simulink model "teste"  (R2012b)
settings: Solver=ode3  StartTime=0.0  StopTime=0.2  FixedStep=1e-6  RelTol=1e-6
undefined symbols (not defined in the file): J, Kd, Ke, Kt, L, P, R
libraries: simulink x40
settings Model: BufferReuse=off  Creator=Juliano  LastModifiedBy=Juliano
settings OptimizationCC: OptimizeBlockIOStorage=off  BufferReuse=off  ExpressionFolding=off  LocalBlockOutputs=off
settings DebuggingCC: SignalInfNanChecking=error  IntegerOverflowMsg=error  ParameterPrecisionLossMsg=none

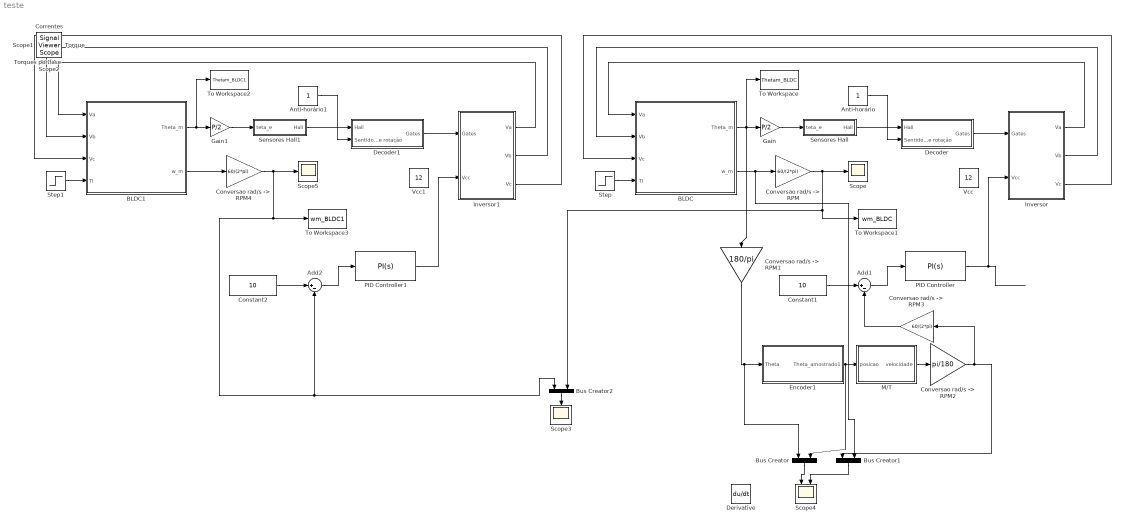
== system teste ==
  Add1 : Sum  Inputs=|+-
  Add2 : Sum  Inputs=|+-
  Anti-horário : Constant
  Anti-horário1 : Constant
  BLDC : Subsystem
  BLDC1 : Subsystem
  Bus Creator : BusCreator  Inputs=2
  Bus Creator1 : BusCreator  Inputs=2
  Bus Creator2 : BusCreator  Inputs=2
  Constant1 : Constant  Value=10
  Constant2 : Constant  Value=10
  "Conversao rad/s -> RPM" : Gain  Gain=60/(2*pi)
  "Conversao rad/s -> RPM1" : Gain  Gain=180/pi
  "Conversao rad/s -> RPM2" : Gain  Gain=pi/180
  "Conversao rad/s -> RPM3" : Gain  Gain=60/(2*pi)
  "Conversao rad/s -> RPM4" : Gain  Gain=60/(2*pi)
  Decoder : Subsystem
  Decoder1 : Subsystem
  Derivative : Derivative
  Encoder1 : Subsystem  mask{Nr=180}
      mask prompts: Nr "Número de pulsos por revolução"
  Gain : Gain  Gain=P/2
  Gain1 : Gain  Gain=P/2
  Inversor : Subsystem
  Inversor1 : Subsystem
  M/T : Subsystem  mask{Ts=0.01/4}
      mask prompts: Ts "Sampling time"
  PID Controller : simulink/Continuous/PID Controller  Controller=PI  TimeDomain=Continuous-time  SampleTime=1  IntegratorMethod=Forward Euler  FilterMethod=Forward Euler  Form=Parallel  P=0.0147690941731554  I=1.64756402232112  D=0  N=100  InitialConditionSource=internal  InitialConditionForIntegrator=8.9768  InitialConditionForFilter=0  ExternalReset=none  ZeroCross=off  LimitOutput=on  UpperSaturationLimit=12  LowerSaturationLimit=-12  LinearizeAsGain=off  AntiWindupMode=none  Kb=1  TrackingMode=off  Kt=1  PParamMin=[ ]  PParamMax=[ ]  IParamMin=[ ]  IParamMax=[ ]  DParamMin=[ ]  DParamMax=[ ]  NParamMin=[ ]  NParamMax=[ ]  KbParamMin=[ ]  KbParamMax=[ ]  KtParamMin=[ ]  KtParamMax=[ ]  POutMin=[ ]  POutMax=[ ]  IOutMin=[ ]  IOutMax=[ ]  DOutMin=[ ]  DOutMax=[ ]  NOutMin=[ ]  NOutMax=[ ]  KbOutMin=[ ]  KbOutMax=[ ]  KtOutMin=[ ]  KtOutMax=[ ]  IntegratorOutMin=[ ]  IntegratorOutMax=[ ]  FilterOutMin=[ ]  FilterOutMax=[ ]  SumOutMin=[ ]  SumOutMax=[ ]  SumI1OutMin=[ ]  SumI1OutMax=[ ]  SumI2OutMin=[ ]  SumI2OutMax=[ ]  SumI3OutMin=[ ]  SumI3OutMax=[ ]  SumDOutMin=[ ]  SumDOutMax=[ ]  SaturationOutMin=[ ]  SaturationOutMax=[ ]  IntegratorContinuousStateAttributes=''  IntegratorStateMustResolveToSignalObject=off  IntegratorRTWStateStorageClass=Auto  FilterContinuousStateAttributes=''  FilterStateMustResolveToSignalObject=off  FilterRTWStateStorageClass=Auto
  PID Controller1 : simulink/Continuous/PID Controller  Controller=PI  TimeDomain=Continuous-time  SampleTime=1  IntegratorMethod=Forward Euler  FilterMethod=Forward Euler  Form=Parallel  P=0.0147690941731554  I=1.64756402232112  D=0  N=100  InitialConditionSource=internal  InitialConditionForIntegrator=8.9768  InitialConditionForFilter=0  ExternalReset=none  ZeroCross=off  LimitOutput=on  UpperSaturationLimit=12  LowerSaturationLimit=-12  LinearizeAsGain=off  AntiWindupMode=none  Kb=1  TrackingMode=off  Kt=1  PParamMin=[ ]  PParamMax=[ ]  IParamMin=[ ]  IParamMax=[ ]  DParamMin=[ ]  DParamMax=[ ]  NParamMin=[ ]  NParamMax=[ ]  KbParamMin=[ ]  KbParamMax=[ ]  KtParamMin=[ ]  KtParamMax=[ ]  POutMin=[ ]  POutMax=[ ]  IOutMin=[ ]  IOutMax=[ ]  DOutMin=[ ]  DOutMax=[ ]  NOutMin=[ ]  NOutMax=[ ]  KbOutMin=[ ]  KbOutMax=[ ]  KtOutMin=[ ]  KtOutMax=[ ]  IntegratorOutMin=[ ]  IntegratorOutMax=[ ]  FilterOutMin=[ ]  FilterOutMax=[ ]  SumOutMin=[ ]  SumOutMax=[ ]  SumI1OutMin=[ ]  SumI1OutMax=[ ]  SumI2OutMin=[ ]  SumI2OutMax=[ ]  SumI3OutMin=[ ]  SumI3OutMax=[ ]  SumDOutMin=[ ]  SumDOutMax=[ ]  SaturationOutMin=[ ]  SaturationOutMax=[ ]  IntegratorContinuousStateAttributes=''  IntegratorStateMustResolveToSignalObject=off  IntegratorRTWStateStorageClass=Auto  FilterContinuousStateAttributes=''  FilterStateMustResolveToSignalObject=off  FilterRTWStateStorageClass=Auto
  Scope : Scope
      settings: TimeRange=0.5  YMin=1100  YMax=3400
  Scope3 : Scope
      settings: TickLabels=on  ShowLegends=on  TimeRange=0.25  YMin=-750  YMax=4250
  Scope4 : Scope  NumInputPorts=2
      settings: TickLabels=on  YMin=900~-75  YMax=2800~425  SaveName=ScopeData7
  Scope5 : Scope
      settings: TimeRange=0.5  YMin=1100  YMax=3400  SaveName=ScopeData9
  Sensores Hall : Subsystem  AncestorBlock=spsPMSynchronousMachineModel/Discrete Trapezoidal/Hall effect sensor
  Sensores Hall1 : Subsystem  AncestorBlock=spsPMSynchronousMachineModel/Discrete Trapezoidal/Hall effect sensor
  Step : Step  Time=0.2  After=0*2e-3  SampleTime=0
  Step1 : Step  Time=0.2  After=0*2e-3  SampleTime=0
  To Workspace : ToWorkspace  VariableName=Thetam_BLDC  SampleTime=-1  SaveFormat=Timeseries
  To Workspace1 : ToWorkspace  VariableName=wm_BLDC  SampleTime=-1  SaveFormat=Timeseries
  To Workspace2 : ToWorkspace  VariableName=Thetam_BLDC1  SampleTime=-1  SaveFormat=Timeseries
  To Workspace3 : ToWorkspace  VariableName=wm_BLDC1  SampleTime=-1  SaveFormat=Timeseries
  Vcc : Constant  Value=12
  Vcc1 : Constant  Value=12
  Correntes : SignalViewerScope  IOType=viewer  NumInputPorts=3  ZoomMode=yonly  RefreshTime=0.035000
      settings: YMin=-5~-5~-5  YMax=5~5~5
  FCEMs : SignalViewerScope  IOType=viewer  NumInputPorts=3  ZoomMode=xonly  RefreshTime=0.035000
      settings: YMin=-5~-5~-5  YMax=5~5~5  SaveName=ScopeData2
  Scope1 : SignalViewerScope  IOType=viewer  RefreshTime=0.035000
      settings: SaveName=ScopeData3
  Scope2 : SignalViewerScope  IOType=viewer  RefreshTime=0.035000
      settings: SaveName=ScopeData4
  Torque : SignalViewerScope  IOType=viewer  ZoomMode=xonly  RefreshTime=0.035000
      settings: SaveToWorkspace=on  SaveName=Torque
  Torques por fase : SignalViewerScope  IOType=viewer  NumInputPorts=3  ZoomMode=xonly  RefreshTime=0.035000
      settings: YMin=-5~-5~-5  YMax=5~5~5
  wires:
  Gain/1 -> Sensores Hall/1(teta_e)
  Sensores Hall/1(Hall) -> Decoder/1("Hall ")
  Decoder/1(Gates) -> Inversor/1(Gates)
  Anti-horário/1 -> Decoder/2(Sentido de rotação)
  Step/1 -> BLDC/4(Tl)
  Inversor/1(Va) -> BLDC/1(Va)
  Inversor/2(Vb) -> BLDC/2(Vb)
  Inversor/3(Vc) -> BLDC/3(Vc)
  BLDC/2(w_m) -> Bus Creator1/2, "Conversao rad/s -> RPM"/1
  "Conversao rad/s -> RPM"/1 -> Bus Creator2/2, To Workspace1/1, Scope/1
  Constant1/1 -> Add1/1
  Add1/1 -> PID Controller/1
  Bus Creator/1 -> Scope4/1
  Bus Creator1/1 -> Scope4/2
  Encoder1/1(Theta_amostrado1) -> M/T/1(posicao), Bus Creator/2
  PID Controller/1 -> Inversor/2(Vcc)
  BLDC/1(Theta_m) -> "Conversao rad/s -> RPM1"/1, Gain/1, To Workspace/1
  M/T/1(velocidade) -> "Conversao rad/s -> RPM2"/1
  "Conversao rad/s -> RPM1"/1 -> Bus Creator/1, Encoder1/1(Theta)
  "Conversao rad/s -> RPM2"/1 -> Bus Creator1/1, "Conversao rad/s -> RPM3"/1
  "Conversao rad/s -> RPM3"/1 -> Add1/2
  Gain1/1 -> Sensores Hall1/1(teta_e)
  Sensores Hall1/1(Hall) -> Decoder1/1("Hall ")
  Decoder1/1(Gates) -> Inversor1/1(Gates)
  Anti-horário1/1 -> Decoder1/2(Sentido de rotação)
  Step1/1 -> BLDC1/4(Tl)
  Inversor1/1(Va) -> BLDC1/1(Va)
  Inversor1/2(Vb) -> BLDC1/2(Vb)
  Inversor1/3(Vc) -> BLDC1/3(Vc)
  BLDC1/2(w_m) -> "Conversao rad/s -> RPM4"/1
  "Conversao rad/s -> RPM4"/1 -> Bus Creator2/1, Add2/2, To Workspace3/1, Scope5/1
  Constant2/1 -> Add2/1
  Add2/1 -> PID Controller1/1
  PID Controller1/1 -> Inversor1/2(Vcc)
  BLDC1/1(Theta_m) -> Gain1/1, To Workspace2/1
  Bus Creator2/1 -> Scope3/1

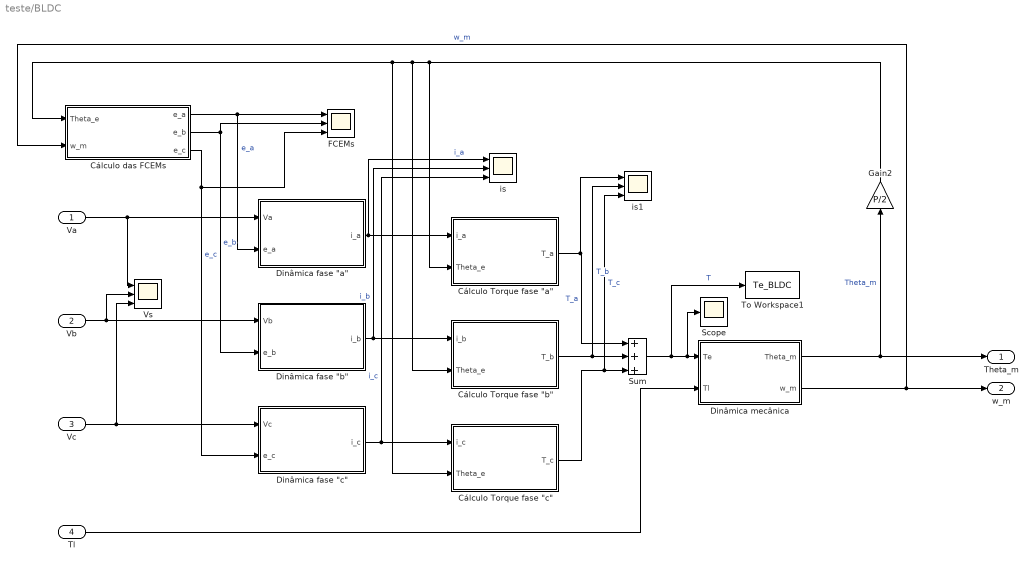
== system teste/BLDC ==
  Va : Inport
  Vb : Inport  Port=2
  Vc : Inport  Port=3
  Tl : Inport  Port=4
  "Cálculo Torque fase \"a\"" : Subsystem
  "Cálculo Torque fase \"b\"" : Subsystem
  "Cálculo Torque fase \"c\"" : Subsystem
  Cálculo das FCEMs : Subsystem
  "Dinâmica fase \"a\"" : Subsystem
  "Dinâmica fase \"b\"" : Subsystem
  "Dinâmica fase \"c\"" : Subsystem
  "Dinâmica mecânica " : Subsystem
  FCEMs : Scope  NumInputPorts=3
      settings: TimeRange=1  YMin=420~-5~-5  YMax=510~5~5  SaveName=ScopeData5
  Gain2 : Gain  Gain=P/2
  Scope : Scope
      settings: TimeRange=1  YMin=420  YMax=510  SaveName=ScopeData4
  Sum : Sum  Inputs=+++
  To Workspace1 : ToWorkspace  VariableName=Te_BLDC  SampleTime=-1  SaveFormat=Timeseries
  Vs : Scope  NumInputPorts=3
      settings: TimeRange=1  YMin=420~-5~-5  YMax=510~5~5  SaveName=ScopeData2
  is : Scope  NumInputPorts=3
      settings: TimeRange=1  YMin=420~-5~-5  YMax=510~5~5  SaveName=ScopeData3
  is1 : Scope  NumInputPorts=3
      settings: TimeRange=1  YMin=420~-5~-5  YMax=510~5~5  SaveName=ScopeData6
  Theta_m : Outport
  w_m : Outport  Port=2
  wires:
  Cálculo das FCEMs/1(e_a) -> FCEMs/1, "Dinâmica fase \"a\""/2(e_a)  "e_a"
  Cálculo das FCEMs/2(e_b) -> "Dinâmica fase \"b\""/2(e_b), FCEMs/2  "e_b"
  Cálculo das FCEMs/3(e_c) -> FCEMs/3, "Dinâmica fase \"c\""/2(e_c)  "e_c"
  Va/1 -> Vs/1, "Dinâmica fase \"a\""/1(Va)
  Vb/1 -> Vs/2, "Dinâmica fase \"b\""/1(Vb)
  Vc/1 -> Vs/3, "Dinâmica fase \"c\""/1(Vc)
  "Dinâmica fase \"a\""/1(i_a) -> is/1, "Cálculo Torque fase \"a\""/1(i_a)  "i_a"
  "Dinâmica fase \"b\""/1(i_b) -> is/2, "Cálculo Torque fase \"b\""/1(i_b)  "i_b"
  "Dinâmica fase \"c\""/1(i_c) -> is/3, "Cálculo Torque fase \"c\""/1(i_c)  "i_c"
  "Cálculo Torque fase \"a\""/1(T_a) -> is1/1, Sum/1  "T_a"
  "Cálculo Torque fase \"b\""/1(T_b) -> is1/2, Sum/2  "T_b"
  "Cálculo Torque fase \"c\""/1(T_c) -> is1/3, Sum/3  "T_c"
  Sum/1 -> To Workspace1/1, Scope/1, "Dinâmica mecânica "/1(Te)  "T"
  "Dinâmica mecânica "/1(Theta_m) -> Theta_m/1, Gain2/1  "Theta_m"
  "Dinâmica mecânica "/2(w_m) -> Cálculo das FCEMs/2(w_m), w_m/1  "w_m"
  Tl/1 -> "Dinâmica mecânica "/2(Tl)
  Gain2/1 -> "Cálculo Torque fase \"a\""/2(Theta_e), "Cálculo Torque fase \"c\""/2(Theta_e), Cálculo das FCEMs/1(Theta_e), "Cálculo Torque fase \"b\""/2(Theta_e)

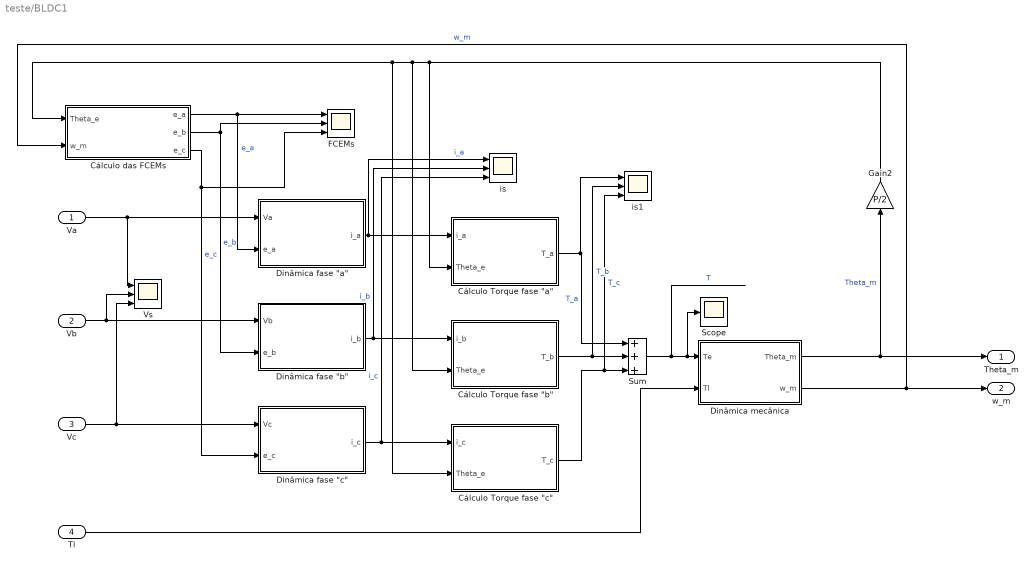
== system teste/BLDC1 ==
  Va : Inport
  Vb : Inport  Port=2
  Vc : Inport  Port=3
  Tl : Inport  Port=4
  "Cálculo Torque fase \"a\"" : Subsystem
  "Cálculo Torque fase \"b\"" : Subsystem
  "Cálculo Torque fase \"c\"" : Subsystem
  Cálculo das FCEMs : Subsystem
  "Dinâmica fase \"a\"" : Subsystem
  "Dinâmica fase \"b\"" : Subsystem
  "Dinâmica fase \"c\"" : Subsystem
  "Dinâmica mecânica " : Subsystem
  FCEMs : Scope  NumInputPorts=3
      settings: TimeRange=1  YMin=420~-5~-5  YMax=510~5~5  SaveName=ScopeData5
  Gain2 : Gain  Gain=P/2
  Scope : Scope
      settings: TimeRange=1  YMin=420  YMax=510  SaveName=ScopeData4
  Sum : Sum  Inputs=+++
  Vs : Scope  NumInputPorts=3
      settings: TimeRange=1  YMin=420~-5~-5  YMax=510~5~5  SaveName=ScopeData2
  is : Scope  NumInputPorts=3
      settings: TimeRange=1  YMin=420~-5~-5  YMax=510~5~5  SaveName=ScopeData3
  is1 : Scope  NumInputPorts=3
      settings: TimeRange=1  YMin=420~-5~-5  YMax=510~5~5  SaveName=ScopeData6
  Theta_m : Outport
  w_m : Outport  Port=2
  wires:
  Cálculo das FCEMs/1(e_a) -> FCEMs/1, "Dinâmica fase \"a\""/2(e_a)  "e_a"
  Cálculo das FCEMs/2(e_b) -> "Dinâmica fase \"b\""/2(e_b), FCEMs/2  "e_b"
  Cálculo das FCEMs/3(e_c) -> FCEMs/3, "Dinâmica fase \"c\""/2(e_c)  "e_c"
  Va/1 -> Vs/1, "Dinâmica fase \"a\""/1(Va)
  Vb/1 -> Vs/2, "Dinâmica fase \"b\""/1(Vb)
  Vc/1 -> Vs/3, "Dinâmica fase \"c\""/1(Vc)
  "Dinâmica fase \"a\""/1(i_a) -> is/1, "Cálculo Torque fase \"a\""/1(i_a)  "i_a"
  "Dinâmica fase \"b\""/1(i_b) -> is/2, "Cálculo Torque fase \"b\""/1(i_b)  "i_b"
  "Dinâmica fase \"c\""/1(i_c) -> is/3, "Cálculo Torque fase \"c\""/1(i_c)  "i_c"
  "Cálculo Torque fase \"a\""/1(T_a) -> is1/1, Sum/1  "T_a"
  "Cálculo Torque fase \"b\""/1(T_b) -> is1/2, Sum/2  "T_b"
  "Cálculo Torque fase \"c\""/1(T_c) -> is1/3, Sum/3  "T_c"
  Sum/1 -> Scope/1, "Dinâmica mecânica "/1(Te)  "T"
  "Dinâmica mecânica "/1(Theta_m) -> Theta_m/1, Gain2/1  "Theta_m"
  "Dinâmica mecânica "/2(w_m) -> Cálculo das FCEMs/2(w_m), w_m/1  "w_m"
  Tl/1 -> "Dinâmica mecânica "/2(Tl)
  Gain2/1 -> "Cálculo Torque fase \"a\""/2(Theta_e), "Cálculo Torque fase \"c\""/2(Theta_e), Cálculo das FCEMs/1(Theta_e), "Cálculo Torque fase \"b\""/2(Theta_e)

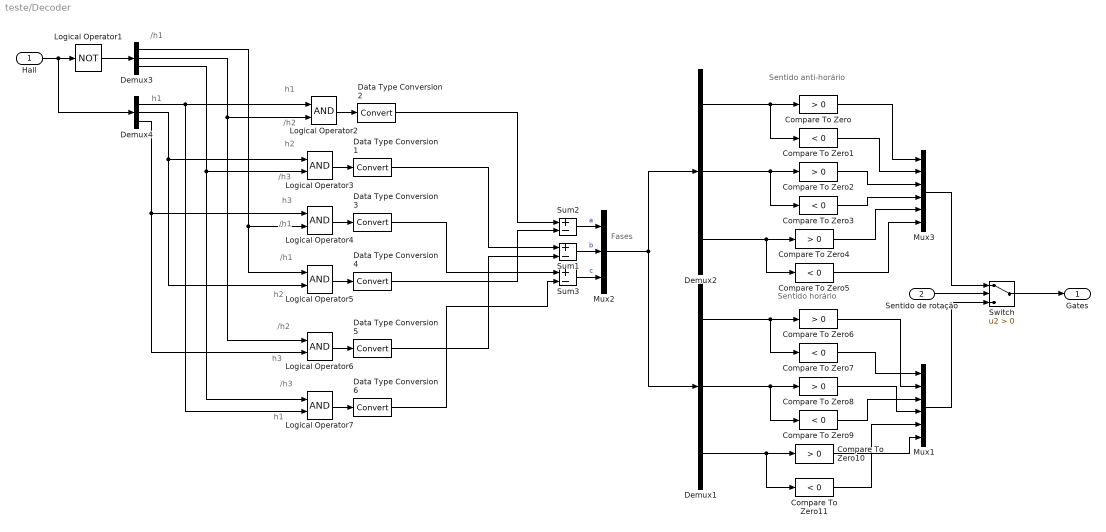
== system teste/Decoder ==
  note: Fases
  note: Sentido horário
  note: Sentido anti-horário
  note: h1
  note: /h3
  note: h3
  note: /h2
  note: h2
  note: /h1
  note: /h1
  note: h3
  note: /h3
  note: h2
  note: /h2
  note: h1
  note: h1
  note: /h1
  "Hall " : Inport
  Sentido de rotação : Inport  Port=2
  Compare To Zero{,2,4,6,8,10} (6 alike) : simulink/Logic and Bit Operations/Compare To Zero  relop=>  OutDataTypeStr=boolean  ZeroCross=off
  Compare To Zero{1,3,5,7,9,11} (6 alike) : simulink/Logic and Bit Operations/Compare To Zero  relop=<  OutDataTypeStr=boolean  ZeroCross=off
  Data Type Conversion{1..6} (6 alike) : DataTypeConversion
  Demux{1..4} (4 alike) : Demux  Outputs=3
  Logical Operator1 : Logic  Operator=NOT  AllPortsSameDT=off  OutDataTypeStr=boolean
  Logical Operator{2..7} (6 alike) : Logic  AllPortsSameDT=off  OutDataTypeStr=boolean
  Mux1 : Mux  Inputs=6
  Mux2 : Mux  Inputs=3
  Mux3 : Mux  Inputs=6
  Sum1 : Sum  Inputs=+-  OutDataTypeStr=double
  Sum2 : Sum  Inputs=+-  OutDataTypeStr=double
  Sum3 : Sum  Inputs=+-  OutDataTypeStr=double
  Switch : Switch  Criteria=u2 > Threshold
  Gates : Outport
  wires:
  Mux2/1 -> Demux1/1, Demux2/1
  Data Type Conversion6/1 -> Sum3/2
  Data Type Conversion3/1 -> Sum3/1
  Data Type Conversion5/1 -> Sum1/2
  Data Type Conversion1/1 -> Sum1/1
  Data Type Conversion4/1 -> Sum2/2
  Data Type Conversion2/1 -> Sum2/1
  Logical Operator7/1 -> Data Type Conversion6/1
  Logical Operator6/1 -> Data Type Conversion5/1
  Logical Operator5/1 -> Data Type Conversion4/1
  Logical Operator4/1 -> Data Type Conversion3/1
  Logical Operator3/1 -> Data Type Conversion1/1
  Sum3/1 -> Mux2/3  "c"
  Sum1/1 -> Mux2/2  "b"
  Sum2/1 -> Mux2/1  "a"
  Logical Operator2/1 -> Data Type Conversion2/1
  Demux3/1 -> Logical Operator5/1, Logical Operator4/2
  Demux3/2 -> Logical Operator6/1, Logical Operator2/2
  Demux3/3 -> Logical Operator7/1, Logical Operator3/2
  Demux4/1 -> Logical Operator7/2, Logical Operator2/1
  Demux4/2 -> Logical Operator5/2, Logical Operator3/1
  Demux4/3 -> Logical Operator6/2, Logical Operator4/1
  Logical Operator1/1 -> Demux3/1
  "Hall "/1 -> Demux4/1, Logical Operator1/1
  Compare To Zero10/1 -> Mux1/6
  Compare To Zero11/1 -> Mux1/5
  Compare To Zero8/1 -> Mux1/4
  Compare To Zero9/1 -> Mux1/3
  Compare To Zero6/1 -> Mux1/2
  Compare To Zero7/1 -> Mux1/1
  Switch/1 -> Gates/1
  Mux1/1 -> Switch/3
  Sentido de rotação/1 -> Switch/2
  Mux3/1 -> Switch/1
  Demux1/3 -> Compare To Zero11/1, Compare To Zero10/1
  Demux1/2 -> Compare To Zero9/1, Compare To Zero8/1
  Demux1/1 -> Compare To Zero7/1, Compare To Zero6/1
  Compare To Zero5/1 -> Mux3/6
  Compare To Zero4/1 -> Mux3/5
  Compare To Zero3/1 -> Mux3/4
  Compare To Zero2/1 -> Mux3/3
  Compare To Zero1/1 -> Mux3/2
  Compare To Zero/1 -> Mux3/1
  Demux2/3 -> Compare To Zero5/1, Compare To Zero4/1
  Demux2/2 -> Compare To Zero3/1, Compare To Zero2/1
  Demux2/1 -> Compare To Zero1/1, Compare To Zero/1

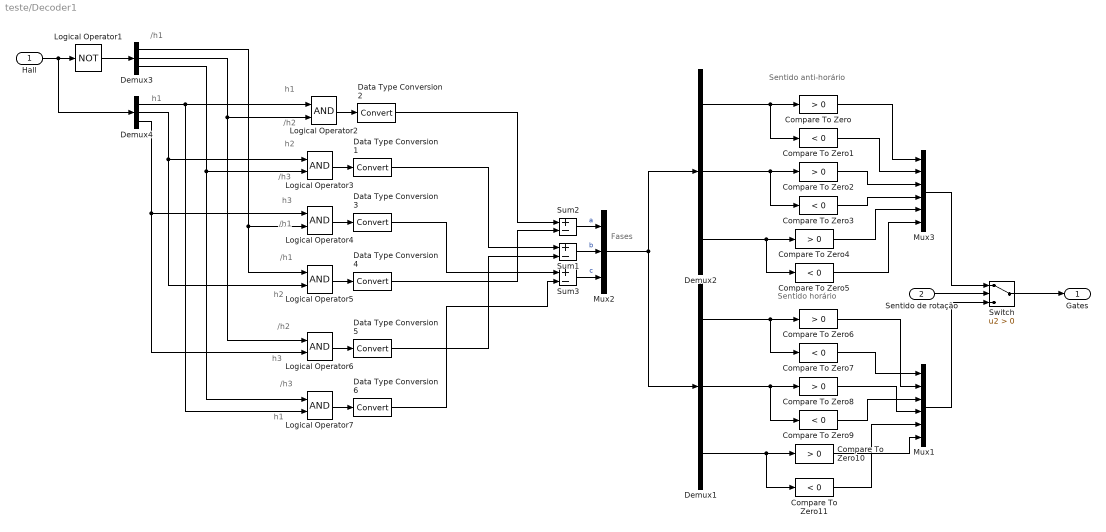
== system teste/Decoder1 ==
  note: Fases
  note: Sentido horário
  note: Sentido anti-horário
  note: h1
  note: /h3
  note: h3
  note: /h2
  note: h2
  note: /h1
  note: /h1
  note: h3
  note: /h3
  note: h2
  note: /h2
  note: h1
  note: h1
  note: /h1
  "Hall " : Inport
  Sentido de rotação : Inport  Port=2
  Compare To Zero{,2,4,6,8,10} (6 alike) : simulink/Logic and Bit Operations/Compare To Zero  relop=>  OutDataTypeStr=boolean  ZeroCross=off
  Compare To Zero{1,3,5,7,9,11} (6 alike) : simulink/Logic and Bit Operations/Compare To Zero  relop=<  OutDataTypeStr=boolean  ZeroCross=off
  Data Type Conversion{1..6} (6 alike) : DataTypeConversion
  Demux{1..4} (4 alike) : Demux  Outputs=3
  Logical Operator1 : Logic  Operator=NOT  AllPortsSameDT=off  OutDataTypeStr=boolean
  Logical Operator{2..7} (6 alike) : Logic  AllPortsSameDT=off  OutDataTypeStr=boolean
  Mux1 : Mux  Inputs=6
  Mux2 : Mux  Inputs=3
  Mux3 : Mux  Inputs=6
  Sum1 : Sum  Inputs=+-  OutDataTypeStr=double
  Sum2 : Sum  Inputs=+-  OutDataTypeStr=double
  Sum3 : Sum  Inputs=+-  OutDataTypeStr=double
  Switch : Switch  Criteria=u2 > Threshold
  Gates : Outport
  wires:
  Mux2/1 -> Demux1/1, Demux2/1
  Data Type Conversion6/1 -> Sum3/2
  Data Type Conversion3/1 -> Sum3/1
  Data Type Conversion5/1 -> Sum1/2
  Data Type Conversion1/1 -> Sum1/1
  Data Type Conversion4/1 -> Sum2/2
  Data Type Conversion2/1 -> Sum2/1
  Logical Operator7/1 -> Data Type Conversion6/1
  Logical Operator6/1 -> Data Type Conversion5/1
  Logical Operator5/1 -> Data Type Conversion4/1
  Logical Operator4/1 -> Data Type Conversion3/1
  Logical Operator3/1 -> Data Type Conversion1/1
  Sum3/1 -> Mux2/3  "c"
  Sum1/1 -> Mux2/2  "b"
  Sum2/1 -> Mux2/1  "a"
  Logical Operator2/1 -> Data Type Conversion2/1
  Demux3/1 -> Logical Operator5/1, Logical Operator4/2
  Demux3/2 -> Logical Operator6/1, Logical Operator2/2
  Demux3/3 -> Logical Operator7/1, Logical Operator3/2
  Demux4/1 -> Logical Operator7/2, Logical Operator2/1
  Demux4/2 -> Logical Operator5/2, Logical Operator3/1
  Demux4/3 -> Logical Operator6/2, Logical Operator4/1
  Logical Operator1/1 -> Demux3/1
  "Hall "/1 -> Demux4/1, Logical Operator1/1
  Compare To Zero10/1 -> Mux1/6
  Compare To Zero11/1 -> Mux1/5
  Compare To Zero8/1 -> Mux1/4
  Compare To Zero9/1 -> Mux1/3
  Compare To Zero6/1 -> Mux1/2
  Compare To Zero7/1 -> Mux1/1
  Switch/1 -> Gates/1
  Mux1/1 -> Switch/3
  Sentido de rotação/1 -> Switch/2
  Mux3/1 -> Switch/1
  Demux1/3 -> Compare To Zero11/1, Compare To Zero10/1
  Demux1/2 -> Compare To Zero9/1, Compare To Zero8/1
  Demux1/1 -> Compare To Zero7/1, Compare To Zero6/1
  Compare To Zero5/1 -> Mux3/6
  Compare To Zero4/1 -> Mux3/5
  Compare To Zero3/1 -> Mux3/4
  Compare To Zero2/1 -> Mux3/3
  Compare To Zero1/1 -> Mux3/2
  Compare To Zero/1 -> Mux3/1
  Demux2/3 -> Compare To Zero5/1, Compare To Zero4/1
  Demux2/2 -> Compare To Zero3/1, Compare To Zero2/1
  Demux2/1 -> Compare To Zero1/1, Compare To Zero/1

== system teste/Encoder1 ==
  note: ATENÇÃO: Para o correto funcionamento desse encoder o step size da simulação deve ser menor do que 360/(4*Nr*Vmax),
      | onde Vmax é o valor máximo da derivada do Theta atigindo durante a simulação
  Theta : Inport
  Bus Creator1 : BusCreator  Inputs=2
  Determinar direçao : Subsystem
  Graus / pulso1 : Gain  Gain=360/(4*Nr)  OutDataTypeStr=double
  Scope3 : Scope
      settings: TimeRange=1  YMin=-1  YMax=1.5  SaveName=ScopeData8
  Sensor Óptico : Subsystem
  Sensor Óptico1 : Subsystem
  Subsystem : Subsystem
  Theta_amostrado1 : Outport
  wires:
  Theta/1 -> Sensor Óptico/1(Theta), Sensor Óptico1/1(Theta)
  Graus / pulso1/1 -> Theta_amostrado1/1
  Subsystem/1(Out) -> Graus / pulso1/1
  Determinar direçao/2(NEG) -> Bus Creator1/2, Subsystem/2(NEG)
  Determinar direçao/1(POS) -> Bus Creator1/1, Subsystem/1(POS)
  Sensor Óptico1/1(Sinal_Pulso) -> Determinar direçao/2(B)  "B"
  Sensor Óptico/1(Sinal_Pulso) -> Determinar direçao/1(A)  "A"
  Bus Creator1/1 -> Scope3/1

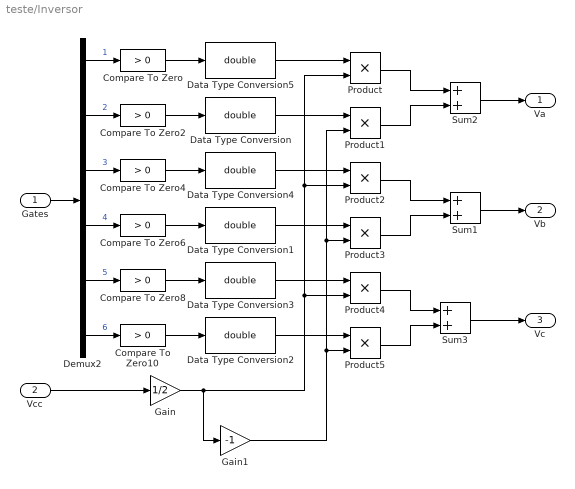
== system teste/Inversor ==
  Gates : Inport
  Vcc : Inport  Port=2
  Compare To Zero : simulink/Logic and Bit Operations/Compare To Zero  relop=>  OutDataTypeStr=uint8  ZeroCross=off
  Compare To Zero{2,6,8,10} (4 alike) : simulink/Logic and Bit Operations/Compare To Zero  relop=>  OutDataTypeStr=boolean  ZeroCross=off
  Compare To Zero4 : simulink/Logic and Bit Operations/Compare To Zero  relop=>  OutDataTypeStr=uint8  ZeroCross=off
  Data Type Conversion{,1..5} (6 alike) : DataTypeConversion  OutDataTypeStr=double
  Demux2 : Demux  Outputs=6
  Gain : Gain  Gain=1/2
  Gain1 : Gain  Gain=-1
  Product{,1..5} (6 alike) : Product  RndMeth=Zero
  Sum1 : Sum  SaturateOnIntegerOverflow=on
  Sum2 : Sum  SaturateOnIntegerOverflow=on
  Sum3 : Sum  SaturateOnIntegerOverflow=on
  Va : Outport
  Vb : Outport  Port=2
  Vc : Outport  Port=3
  wires:
  Vcc/1 -> Gain/1
  Sum1/1 -> Vb/1
  Sum3/1 -> Vc/1
  Sum2/1 -> Va/1
  Gates/1 -> Demux2/1
  Demux2/1 -> Compare To Zero/1  "1"
  Demux2/2 -> Compare To Zero2/1  "2"
  Demux2/3 -> Compare To Zero4/1  "3"
  Demux2/4 -> Compare To Zero6/1  "4"
  Demux2/5 -> Compare To Zero8/1  "5"
  Demux2/6 -> Compare To Zero10/1  "6"
  Compare To Zero/1 -> Data Type Conversion5/1
  Compare To Zero2/1 -> Data Type Conversion/1
  Compare To Zero4/1 -> Data Type Conversion4/1
  Compare To Zero6/1 -> Data Type Conversion1/1
  Compare To Zero8/1 -> Data Type Conversion3/1
  Compare To Zero10/1 -> Data Type Conversion2/1
  Product/1 -> Sum2/1
  Product1/1 -> Sum2/2
  Product2/1 -> Sum1/1
  Product3/1 -> Sum1/2
  Product4/1 -> Sum3/1
  Product5/1 -> Sum3/2
  Data Type Conversion2/1 -> Product5/1
  Data Type Conversion3/1 -> Product4/1
  Data Type Conversion1/1 -> Product3/1
  Data Type Conversion4/1 -> Product2/1
  Data Type Conversion/1 -> Product1/1
  Data Type Conversion5/1 -> Product/1
  Gain1/1 -> Product5/2, Product3/2, Product1/2
  Gain/1 -> Gain1/1, Product4/2, Product2/2, Product/2

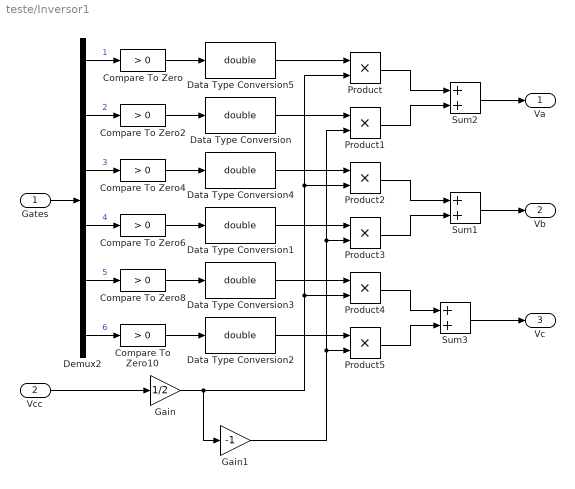
== system teste/Inversor1 ==
  Gates : Inport
  Vcc : Inport  Port=2
  Compare To Zero : simulink/Logic and Bit Operations/Compare To Zero  relop=>  OutDataTypeStr=uint8  ZeroCross=off
  Compare To Zero{2,6,8,10} (4 alike) : simulink/Logic and Bit Operations/Compare To Zero  relop=>  OutDataTypeStr=boolean  ZeroCross=off
  Compare To Zero4 : simulink/Logic and Bit Operations/Compare To Zero  relop=>  OutDataTypeStr=uint8  ZeroCross=off
  Data Type Conversion{,1..5} (6 alike) : DataTypeConversion  OutDataTypeStr=double
  Demux2 : Demux  Outputs=6
  Gain : Gain  Gain=1/2
  Gain1 : Gain  Gain=-1
  Product{,1..5} (6 alike) : Product  RndMeth=Zero
  Sum1 : Sum  SaturateOnIntegerOverflow=on
  Sum2 : Sum  SaturateOnIntegerOverflow=on
  Sum3 : Sum  SaturateOnIntegerOverflow=on
  Va : Outport
  Vb : Outport  Port=2
  Vc : Outport  Port=3
  wires:
  Vcc/1 -> Gain/1
  Sum1/1 -> Vb/1
  Sum3/1 -> Vc/1
  Sum2/1 -> Va/1
  Gates/1 -> Demux2/1
  Demux2/1 -> Compare To Zero/1  "1"
  Demux2/2 -> Compare To Zero2/1  "2"
  Demux2/3 -> Compare To Zero4/1  "3"
  Demux2/4 -> Compare To Zero6/1  "4"
  Demux2/5 -> Compare To Zero8/1  "5"
  Demux2/6 -> Compare To Zero10/1  "6"
  Compare To Zero/1 -> Data Type Conversion5/1
  Compare To Zero2/1 -> Data Type Conversion/1
  Compare To Zero4/1 -> Data Type Conversion4/1
  Compare To Zero6/1 -> Data Type Conversion1/1
  Compare To Zero8/1 -> Data Type Conversion3/1
  Compare To Zero10/1 -> Data Type Conversion2/1
  Product/1 -> Sum2/1
  Product1/1 -> Sum2/2
  Product2/1 -> Sum1/1
  Product3/1 -> Sum1/2
  Product4/1 -> Sum3/1
  Product5/1 -> Sum3/2
  Data Type Conversion2/1 -> Product5/1
  Data Type Conversion3/1 -> Product4/1
  Data Type Conversion1/1 -> Product3/1
  Data Type Conversion4/1 -> Product2/1
  Data Type Conversion/1 -> Product1/1
  Data Type Conversion5/1 -> Product/1
  Gain1/1 -> Product5/2, Product3/2, Product1/2
  Gain/1 -> Gain1/1, Product4/2, Product2/2, Product/2

== system teste/M//T ==
  note: pode ser que as memórias 0 e 1 atualizem antes da 2....
  posicao : Inport
  Clock : Clock
  Compare To Constant : simulink/Logic and Bit Operations/Compare To Constant  relop=>=  const=Ts  OutDataTypeStr=boolean
  Detect Change : simulink/Logic and Bit Operations/Detect Change  vinit=0  InputProcessing=Inherited  OutDataTypeStr=boolean
  Divide : Product  Inputs=*/
  Logical Operator : Logic  AllPortsSameDT=off  OutDataTypeStr=boolean
  Memória controlavel : Subsystem
  Memória controlavel1 : Subsystem
  Memória controlavel2 : Subsystem
  Sum : Sum  Inputs=+-|
  Sum1 : Sum  Inputs=+-|
  velocidade : Outport
  wires:
  Memória controlavel2/1(Out) -> velocidade/1
  Logical Operator/1 -> Memória controlavel2/2(ctrl), Memória controlavel/2(ctrl), Memória controlavel1/2(ctrl)
  Detect Change/1 -> Logical Operator/1
  Compare To Constant/1 -> Logical Operator/2
  Sum/1 -> Divide/1
  Memória controlavel1/1(Out) -> Sum1/2
  Clock/1 -> Sum1/1, Memória controlavel1/1(In)
  Divide/1 -> Memória controlavel2/1(In)
  Memória controlavel/1(Out) -> Sum/2
  Sum1/1 -> Divide/2, Compare To Constant/1
  posicao/1 -> Memória controlavel/1(In), Sum/1, Detect Change/1

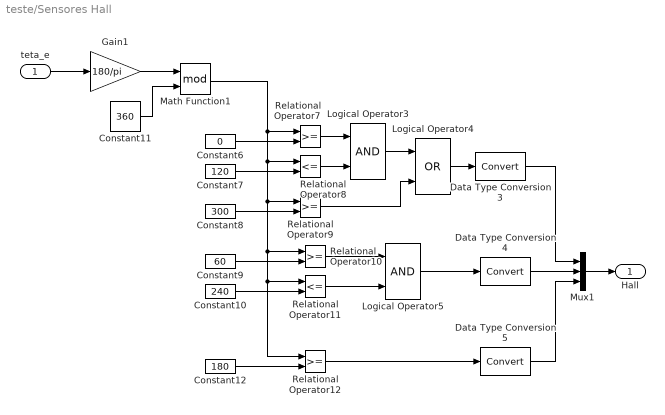
== system teste/Sensores Hall ==
  teta_e : Inport
  Constant10 : Constant  Value=240
  Constant11 : Constant  Value=360
  Constant12 : Constant  Value=180
  Constant6 : Constant  Value=0
  Constant7 : Constant  Value=120
  Constant8 : Constant  Value=300
  Constant9 : Constant  Value=60
  Data Type Conversion3 : DataTypeConversion  SaturateOnIntegerOverflow=on  RndMeth=Zero
  Data Type Conversion4 : DataTypeConversion  SaturateOnIntegerOverflow=on  RndMeth=Zero
  Data Type Conversion5 : DataTypeConversion  SaturateOnIntegerOverflow=on  RndMeth=Zero
  Gain1 : Gain  Gain=180/pi
  Logical Operator3 : Logic  AllPortsSameDT=off  OutDataTypeStr=boolean
  Logical Operator4 : Logic  Operator=OR  AllPortsSameDT=off  OutDataTypeStr=boolean
  Logical Operator5 : Logic  AllPortsSameDT=off  OutDataTypeStr=boolean
  Math Function1 : Math  Operator=mod  SaturateOnIntegerOverflow=on
  Mux1 : Mux  Inputs=3
  Relational Operator{7,9..10,12} (4 alike) : RelationalOperator  InputSameDT=on
  Relational Operator11 : RelationalOperator  Operator=<=  InputSameDT=on
  Relational Operator8 : RelationalOperator  Operator=<=  InputSameDT=on
  Hall : Outport
  wires:
  teta_e/1 -> Gain1/1
  Constant6/1 -> Relational Operator7/2
  Constant7/1 -> Relational Operator8/2
  Constant8/1 -> Relational Operator9/2
  Relational Operator9/1 -> Logical Operator4/2
  Logical Operator3/1 -> Logical Operator4/1
  Relational Operator7/1 -> Logical Operator3/1
  Relational Operator8/1 -> Logical Operator3/2
  Relational Operator10/1 -> Logical Operator5/1
  Relational Operator11/1 -> Logical Operator5/2
  Constant9/1 -> Relational Operator10/2
  Constant10/1 -> Relational Operator11/2
  Constant12/1 -> Relational Operator12/2
  Mux1/1 -> Hall/1
  Data Type Conversion3/1 -> Mux1/1
  Data Type Conversion4/1 -> Mux1/2
  Data Type Conversion5/1 -> Mux1/3
  Logical Operator4/1 -> Data Type Conversion3/1
  Logical Operator5/1 -> Data Type Conversion4/1
  Relational Operator12/1 -> Data Type Conversion5/1
  Gain1/1 -> Math Function1/1
  Constant11/1 -> Math Function1/2
  Math Function1/1 -> Relational Operator8/1, Relational Operator9/1, Relational Operator10/1, Relational Operator11/1, Relational Operator12/1, Relational Operator7/1

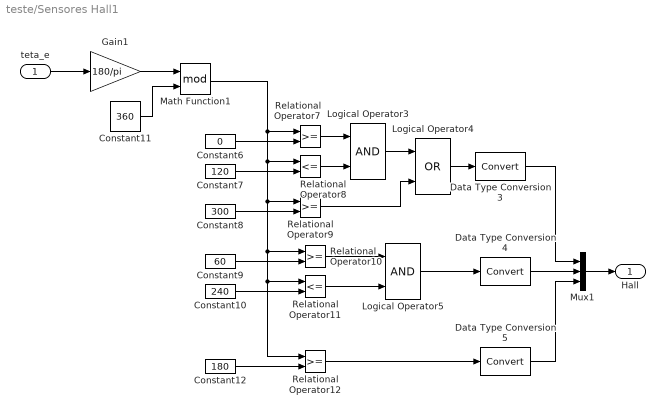
== system teste/Sensores Hall1 ==
  teta_e : Inport
  Constant10 : Constant  Value=240
  Constant11 : Constant  Value=360
  Constant12 : Constant  Value=180
  Constant6 : Constant  Value=0
  Constant7 : Constant  Value=120
  Constant8 : Constant  Value=300
  Constant9 : Constant  Value=60
  Data Type Conversion3 : DataTypeConversion  SaturateOnIntegerOverflow=on  RndMeth=Zero
  Data Type Conversion4 : DataTypeConversion  SaturateOnIntegerOverflow=on  RndMeth=Zero
  Data Type Conversion5 : DataTypeConversion  SaturateOnIntegerOverflow=on  RndMeth=Zero
  Gain1 : Gain  Gain=180/pi
  Logical Operator3 : Logic  AllPortsSameDT=off  OutDataTypeStr=boolean
  Logical Operator4 : Logic  Operator=OR  AllPortsSameDT=off  OutDataTypeStr=boolean
  Logical Operator5 : Logic  AllPortsSameDT=off  OutDataTypeStr=boolean
  Math Function1 : Math  Operator=mod  SaturateOnIntegerOverflow=on
  Mux1 : Mux  Inputs=3
  Relational Operator{7,9..10,12} (4 alike) : RelationalOperator  InputSameDT=on
  Relational Operator11 : RelationalOperator  Operator=<=  InputSameDT=on
  Relational Operator8 : RelationalOperator  Operator=<=  InputSameDT=on
  Hall : Outport
  wires:
  teta_e/1 -> Gain1/1
  Constant6/1 -> Relational Operator7/2
  Constant7/1 -> Relational Operator8/2
  Constant8/1 -> Relational Operator9/2
  Relational Operator9/1 -> Logical Operator4/2
  Logical Operator3/1 -> Logical Operator4/1
  Relational Operator7/1 -> Logical Operator3/1
  Relational Operator8/1 -> Logical Operator3/2
  Relational Operator10/1 -> Logical Operator5/1
  Relational Operator11/1 -> Logical Operator5/2
  Constant9/1 -> Relational Operator10/2
  Constant10/1 -> Relational Operator11/2
  Constant12/1 -> Relational Operator12/2
  Mux1/1 -> Hall/1
  Data Type Conversion3/1 -> Mux1/1
  Data Type Conversion4/1 -> Mux1/2
  Data Type Conversion5/1 -> Mux1/3
  Logical Operator4/1 -> Data Type Conversion3/1
  Logical Operator5/1 -> Data Type Conversion4/1
  Relational Operator12/1 -> Data Type Conversion5/1
  Gain1/1 -> Math Function1/1
  Constant11/1 -> Math Function1/2
  Math Function1/1 -> Relational Operator8/1, Relational Operator9/1, Relational Operator10/1, Relational Operator11/1, Relational Operator12/1, Relational Operator7/1

== system teste/BLDC/Cálculo Torque fase "a" ==
  i_a : Inport
  Theta_e : Inport  Port=2
  Constant1 : Constant  Value=360
  Gain : Gain  Gain=Kt/2
  Gain1 : Gain  Gain=180/pi
  Math Function1 : Math  Operator=mod  SaturateOnIntegerOverflow=on
  Product : Product  RndMeth=Zero
  fa1 : Lookup  InputValues=[0 30 60 90 120 150 180 210 240 270 300 330 360]  Table=[ 1 1 1 0 -1 -1 -1 -1 -1 0 1 1 1]
  T_a : Outport
  wires:
  i_a/1 -> Gain/1
  Gain/1 -> Product/2
  Math Function1/1 -> fa1/1
  Theta_e/1 -> Gain1/1
  fa1/1 -> Product/1
  Product/1 -> T_a/1
  Gain1/1 -> Math Function1/1
  Constant1/1 -> Math Function1/2

== system teste/BLDC/Cálculo Torque fase "b" ==
  i_b : Inport
  Theta_e : Inport  Port=2
  Constant1 : Constant  Value=360
  Gain : Gain  Gain=Kt/2
  Gain1 : Gain  Gain=180/pi
  Math Function1 : Math  Operator=mod  SaturateOnIntegerOverflow=on
  Product : Product  RndMeth=Zero
  fb2 : Lookup  InputValues=[0 30 60 90 120 150 180 210 240 270 300 330 360]  Table=[-1 0 1 1 1 1 1 0 -1 -1 -1 -1 -1]
  T_b : Outport
  wires:
  Product/1 -> T_b/1
  fb2/1 -> Product/1
  Theta_e/1 -> Gain1/1
  Math Function1/1 -> fb2/1
  Gain/1 -> Product/2
  i_b/1 -> Gain/1
  Gain1/1 -> Math Function1/1
  Constant1/1 -> Math Function1/2

== system teste/BLDC/Cálculo Torque fase "c" ==
  i_c : Inport
  Theta_e : Inport  Port=2
  Constant1 : Constant  Value=360
  Gain : Gain  Gain=Kt/2
  Gain1 : Gain  Gain=180/pi
  Math Function1 : Math  Operator=mod  SaturateOnIntegerOverflow=on
  Product : Product  RndMeth=Zero
  fc1 : Lookup  InputValues=[0 30 60 90 120 150 180 210 240 270 300 330 360]  Table=[-1 -1 -1 -1 -1 0 1 1 1 1 1 0 -1]
  T_c : Outport
  wires:
  i_c/1 -> Gain/1
  Gain/1 -> Product/2
  Math Function1/1 -> fc1/1
  Theta_e/1 -> Gain1/1
  fc1/1 -> Product/1
  Product/1 -> T_c/1
  Gain1/1 -> Math Function1/1
  Constant1/1 -> Math Function1/2

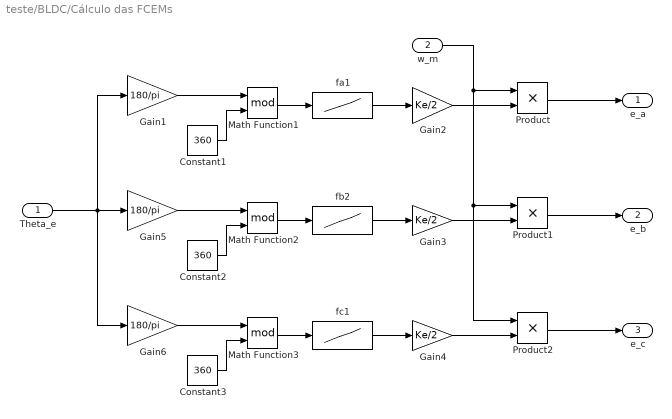
== system teste/BLDC/Cálculo das FCEMs ==
  Theta_e : Inport
  w_m : Inport  Port=2
  Constant1 : Constant  Value=360
  Constant2 : Constant  Value=360
  Constant3 : Constant  Value=360
  Gain1 : Gain  Gain=180/pi
  Gain2 : Gain  Gain=Ke/2
  Gain3 : Gain  Gain=Ke/2
  Gain4 : Gain  Gain=Ke/2
  Gain5 : Gain  Gain=180/pi
  Gain6 : Gain  Gain=180/pi
  Math Function1 : Math  Operator=mod  SaturateOnIntegerOverflow=on
  Math Function2 : Math  Operator=mod  SaturateOnIntegerOverflow=on
  Math Function3 : Math  Operator=mod  SaturateOnIntegerOverflow=on
  Product : Product  RndMeth=Zero
  Product1 : Product  RndMeth=Zero
  Product2 : Product  RndMeth=Zero
  fa1 : Lookup  InputValues=[0 30 60 90 120 150 180 210 240 270 300 330 360]  Table=[ 1 1 1 0 -1 -1 -1 -1 -1 0 1 1 1]
  fb2 : Lookup  InputValues=[0 30 60 90 120 150 180 210 240 270 300 330 360]  Table=[-1 0 1 1 1 1 1 0 -1 -1 -1 -1 -1]
  fc1 : Lookup  InputValues=[0 30 60 90 120 150 180 210 240 270 300 330 360]  Table=[-1 -1 -1 -1 -1 0 1 1 1 1 1 0 -1]
  e_a : Outport
  e_b : Outport  Port=2
  e_c : Outport  Port=3
  wires:
  fc1/1 -> Gain4/1
  Math Function3/1 -> fc1/1
  fb2/1 -> Gain3/1
  Math Function2/1 -> fb2/1
  fa1/1 -> Gain2/1
  Math Function1/1 -> fa1/1
  Gain6/1 -> Math Function3/1
  Gain5/1 -> Math Function2/1
  Gain1/1 -> Math Function1/1
  Gain4/1 -> Product2/2
  Gain3/1 -> Product1/2
  w_m/1 -> Product2/1, Product1/1, Product/1
  Gain2/1 -> Product/2
  Product2/1 -> e_c/1
  Theta_e/1 -> Gain6/1, Gain1/1, Gain5/1
  Product1/1 -> e_b/1
  Product/1 -> e_a/1
  Constant1/1 -> Math Function1/2
  Constant2/1 -> Math Function2/2
  Constant3/1 -> Math Function3/2

== system teste/BLDC/Dinâmica fase "a" ==
  note: Gain
  Va : Inport
  e_a : Inport  Port=2
  " " : Gain  Gain=1/L
  Gain : Gain  Gain=R
  Integrator : Integrator
  Sum : Sum  Inputs=+--
  i_a : Outport
  wires:
  Integrator/1 -> i_a/1, Gain/1
  Va/1 -> Sum/1
  Sum/1 -> " "/1
  " "/1 -> Integrator/1
  Gain/1 -> Sum/3
  e_a/1 -> Sum/2

== system teste/BLDC/Dinâmica fase "b" ==
  note: Gain
  Vb : Inport
  e_b : Inport  Port=2
  " " : Gain  Gain=1/L
  Gain : Gain  Gain=R
  Integrator : Integrator
  Sum : Sum  Inputs=+--
  i_b : Outport
  wires:
  e_b/1 -> Sum/2
  Gain/1 -> Sum/3
  " "/1 -> Integrator/1
  Sum/1 -> " "/1
  Vb/1 -> Sum/1
  Integrator/1 -> Gain/1, i_b/1

== system teste/BLDC/Dinâmica fase "c" ==
  note: Gain
  Vc : Inport
  e_c : Inport  Port=2
  " " : Gain  Gain=1/L
  Gain : Gain  Gain=R
  Integrator : Integrator
  Sum : Sum  Inputs=+--
  i_c : Outport
  wires:
  Integrator/1 -> i_c/1, Gain/1
  Vc/1 -> Sum/1
  Sum/1 -> " "/1
  " "/1 -> Integrator/1
  Gain/1 -> Sum/3
  e_c/1 -> Sum/2

== system teste/BLDC/Dinâmica mecânica  ==
  Te : Inport
  Tl : Inport  Port=2
  Gain : Gain  Gain=1/J
  Gain1 : Gain  Gain=Kd
  Integrator : Integrator
  Integrator1 : Integrator
  Sum1 : Sum  Inputs=+--
  Theta_m : Outport
  w_m : Outport  Port=2
  wires:
  Sum1/1 -> Gain/1
  Gain/1 -> Integrator/1
  Integrator/1 -> w_m/1, Integrator1/1, Gain1/1
  Te/1 -> Sum1/1
  Gain1/1 -> Sum1/3
  Tl/1 -> Sum1/2
  Integrator1/1 -> Theta_m/1

== system teste/BLDC1/Cálculo Torque fase "a" ==
  i_a : Inport
  Theta_e : Inport  Port=2
  Constant1 : Constant  Value=360
  Gain : Gain  Gain=Kt/2
  Gain1 : Gain  Gain=180/pi
  Math Function1 : Math  Operator=mod  SaturateOnIntegerOverflow=on
  Product : Product  RndMeth=Zero
  fa1 : Lookup  InputValues=[0 30 60 90 120 150 180 210 240 270 300 330 360]  Table=[ 1 1 1 0 -1 -1 -1 -1 -1 0 1 1 1]
  T_a : Outport
  wires:
  i_a/1 -> Gain/1
  Gain/1 -> Product/2
  Math Function1/1 -> fa1/1
  Theta_e/1 -> Gain1/1
  fa1/1 -> Product/1
  Product/1 -> T_a/1
  Gain1/1 -> Math Function1/1
  Constant1/1 -> Math Function1/2

== system teste/BLDC1/Cálculo Torque fase "b" ==
  i_b : Inport
  Theta_e : Inport  Port=2
  Constant1 : Constant  Value=360
  Gain : Gain  Gain=Kt/2
  Gain1 : Gain  Gain=180/pi
  Math Function1 : Math  Operator=mod  SaturateOnIntegerOverflow=on
  Product : Product  RndMeth=Zero
  fb2 : Lookup  InputValues=[0 30 60 90 120 150 180 210 240 270 300 330 360]  Table=[-1 0 1 1 1 1 1 0 -1 -1 -1 -1 -1]
  T_b : Outport
  wires:
  Product/1 -> T_b/1
  fb2/1 -> Product/1
  Theta_e/1 -> Gain1/1
  Math Function1/1 -> fb2/1
  Gain/1 -> Product/2
  i_b/1 -> Gain/1
  Gain1/1 -> Math Function1/1
  Constant1/1 -> Math Function1/2

== system teste/BLDC1/Cálculo Torque fase "c" ==
  i_c : Inport
  Theta_e : Inport  Port=2
  Constant1 : Constant  Value=360
  Gain : Gain  Gain=Kt/2
  Gain1 : Gain  Gain=180/pi
  Math Function1 : Math  Operator=mod  SaturateOnIntegerOverflow=on
  Product : Product  RndMeth=Zero
  fc1 : Lookup  InputValues=[0 30 60 90 120 150 180 210 240 270 300 330 360]  Table=[-1 -1 -1 -1 -1 0 1 1 1 1 1 0 -1]
  T_c : Outport
  wires:
  i_c/1 -> Gain/1
  Gain/1 -> Product/2
  Math Function1/1 -> fc1/1
  Theta_e/1 -> Gain1/1
  fc1/1 -> Product/1
  Product/1 -> T_c/1
  Gain1/1 -> Math Function1/1
  Constant1/1 -> Math Function1/2

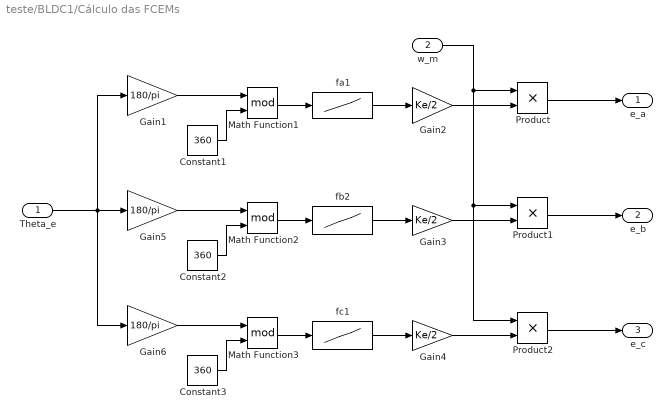
== system teste/BLDC1/Cálculo das FCEMs ==
  Theta_e : Inport
  w_m : Inport  Port=2
  Constant1 : Constant  Value=360
  Constant2 : Constant  Value=360
  Constant3 : Constant  Value=360
  Gain1 : Gain  Gain=180/pi
  Gain2 : Gain  Gain=Ke/2
  Gain3 : Gain  Gain=Ke/2
  Gain4 : Gain  Gain=Ke/2
  Gain5 : Gain  Gain=180/pi
  Gain6 : Gain  Gain=180/pi
  Math Function1 : Math  Operator=mod  SaturateOnIntegerOverflow=on
  Math Function2 : Math  Operator=mod  SaturateOnIntegerOverflow=on
  Math Function3 : Math  Operator=mod  SaturateOnIntegerOverflow=on
  Product : Product  RndMeth=Zero
  Product1 : Product  RndMeth=Zero
  Product2 : Product  RndMeth=Zero
  fa1 : Lookup  InputValues=[0 30 60 90 120 150 180 210 240 270 300 330 360]  Table=[ 1 1 1 0 -1 -1 -1 -1 -1 0 1 1 1]
  fb2 : Lookup  InputValues=[0 30 60 90 120 150 180 210 240 270 300 330 360]  Table=[-1 0 1 1 1 1 1 0 -1 -1 -1 -1 -1]
  fc1 : Lookup  InputValues=[0 30 60 90 120 150 180 210 240 270 300 330 360]  Table=[-1 -1 -1 -1 -1 0 1 1 1 1 1 0 -1]
  e_a : Outport
  e_b : Outport  Port=2
  e_c : Outport  Port=3
  wires:
  fc1/1 -> Gain4/1
  Math Function3/1 -> fc1/1
  fb2/1 -> Gain3/1
  Math Function2/1 -> fb2/1
  fa1/1 -> Gain2/1
  Math Function1/1 -> fa1/1
  Gain6/1 -> Math Function3/1
  Gain5/1 -> Math Function2/1
  Gain1/1 -> Math Function1/1
  Gain4/1 -> Product2/2
  Gain3/1 -> Product1/2
  w_m/1 -> Product2/1, Product1/1, Product/1
  Gain2/1 -> Product/2
  Product2/1 -> e_c/1
  Theta_e/1 -> Gain6/1, Gain1/1, Gain5/1
  Product1/1 -> e_b/1
  Product/1 -> e_a/1
  Constant1/1 -> Math Function1/2
  Constant2/1 -> Math Function2/2
  Constant3/1 -> Math Function3/2

== system teste/BLDC1/Dinâmica fase "a" ==
  note: Gain
  Va : Inport
  e_a : Inport  Port=2
  " " : Gain  Gain=1/L
  Gain : Gain  Gain=R
  Integrator : Integrator
  Sum : Sum  Inputs=+--
  i_a : Outport
  wires:
  Integrator/1 -> i_a/1, Gain/1
  Va/1 -> Sum/1
  Sum/1 -> " "/1
  " "/1 -> Integrator/1
  Gain/1 -> Sum/3
  e_a/1 -> Sum/2

== system teste/BLDC1/Dinâmica fase "b" ==
  note: Gain
  Vb : Inport
  e_b : Inport  Port=2
  " " : Gain  Gain=1/L
  Gain : Gain  Gain=R
  Integrator : Integrator
  Sum : Sum  Inputs=+--
  i_b : Outport
  wires:
  e_b/1 -> Sum/2
  Gain/1 -> Sum/3
  " "/1 -> Integrator/1
  Sum/1 -> " "/1
  Vb/1 -> Sum/1
  Integrator/1 -> Gain/1, i_b/1

== system teste/BLDC1/Dinâmica fase "c" ==
  note: Gain
  Vc : Inport
  e_c : Inport  Port=2
  " " : Gain  Gain=1/L
  Gain : Gain  Gain=R
  Integrator : Integrator
  Sum : Sum  Inputs=+--
  i_c : Outport
  wires:
  Integrator/1 -> i_c/1, Gain/1
  Vc/1 -> Sum/1
  Sum/1 -> " "/1
  " "/1 -> Integrator/1
  Gain/1 -> Sum/3
  e_c/1 -> Sum/2

== system teste/BLDC1/Dinâmica mecânica  ==
  Te : Inport
  Tl : Inport  Port=2
  Gain : Gain  Gain=1/J
  Gain1 : Gain  Gain=Kd
  Integrator : Integrator
  Integrator1 : Integrator
  Sum1 : Sum  Inputs=+--
  Theta_m : Outport
  w_m : Outport  Port=2
  wires:
  Sum1/1 -> Gain/1
  Gain/1 -> Integrator/1
  Integrator/1 -> w_m/1, Integrator1/1, Gain1/1
  Te/1 -> Sum1/1
  Gain1/1 -> Sum1/3
  Tl/1 -> Sum1/2
  Integrator1/1 -> Theta_m/1

== system teste/Encoder1/Determinar direçao ==
  note: Dependendo dos valores passados e dos valores atuais
      | dos pulsos de cada sensor óptico, determina o sentido
      | de rotaçao.
  note: 00
      | 01
      | 10
      | 11
  note: 00 01 10 11
  note: 0	-	+	0
      | +	0	0	-
      | -	0	0	+
      | 0	+	-	0
  note: Implementa a seguinte tabela verdade:
  note: AB
  note: A'B'
  note: A,B = Valores atuais dos sinais A e B
      | A'B' = Valores passados do sinais A e B
  A : Inport
  B : Inport  Port=2
  Bus Creator1 : BusCreator
  Combinatorial  Logic : CombinatorialLogic  TruthTable=[ 0 0 ; 0 1 ; 1 0 ; 0 0 ; 1 0 ; 0 0 ; 0 0 ; 0 1 ; 0 1 ; 0 0 ; 0 0 ; 1 0 ; 0 0 ; 1 0 ; 0 1 ; 0 0]
  Demux : Demux  Outputs=2
  Memory : Memory
  Memory1 : Memory
  POS : Outport
  NEG : Outport  Port=2
  wires:
  B/1 -> Bus Creator1/4, Memory1/1
  Memory1/1 -> Bus Creator1/2
  Bus Creator1/1 -> Combinatorial  Logic/1
  Memory/1 -> Bus Creator1/1
  Combinatorial  Logic/1 -> Demux/1
  Demux/2 -> NEG/1
  A/1 -> Bus Creator1/3, Memory/1
  Demux/1 -> POS/1

== system teste/Encoder1/Sensor Óptico ==
  note: Saída do sensor óptico é:
      | 1, se	0 < mod(T,Tp) < Tp/2
      |  0, se      Tp/2 < mod(T,Tp) < Tp
  Theta : Inport
  Constant : Constant  Value=0
  Constant1 : Constant  Value=Nr
  Constant2 : Constant  Value=360
  Divide : Product  Inputs=*/
  Gain : Gain  Gain=1/2
  Logical Operator : Logic  AllPortsSameDT=off  OutDataTypeStr=boolean
  Math Function : Math  Operator=mod  SaturateOnIntegerOverflow=on
  Relational Operator : RelationalOperator  Operator=>  OutDataTypeStr=boolean
  Relational Operator1 : RelationalOperator  Operator=<  OutDataTypeStr=boolean
  Sinal_Pulso : Outport
  wires:
  Constant1/1 -> Divide/2
  Constant2/1 -> Divide/1
  Logical Operator/1 -> Sinal_Pulso/1
  Gain/1 -> Relational Operator1/2
  Divide/1 -> Gain/1, Math Function/2  "Theta_p"
  Constant/1 -> Relational Operator/2
  Relational Operator1/1 -> Logical Operator/2
  Relational Operator/1 -> Logical Operator/1
  Theta/1 -> Math Function/1
  Math Function/1 -> Relational Operator/1, Relational Operator1/1

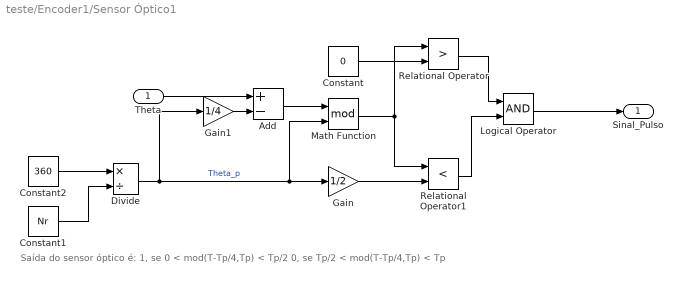
== system teste/Encoder1/Sensor Óptico1 ==
  note: Saída do sensor óptico é:
      | 1, se	0 < mod(T-Tp/4,Tp) < Tp/2
      |  0, se     Tp/2 < mod(T-Tp/4,Tp) < Tp
  Theta : Inport
  Add : Sum  Inputs=+-
  Constant : Constant  Value=0
  Constant1 : Constant  Value=Nr
  Constant2 : Constant  Value=360
  Divide : Product  Inputs=*/
  Gain : Gain  Gain=1/2
  Gain1 : Gain  Gain=1/4
  Logical Operator : Logic  AllPortsSameDT=off  OutDataTypeStr=boolean
  Math Function : Math  Operator=mod  SaturateOnIntegerOverflow=on
  Relational Operator : RelationalOperator  Operator=>  OutDataTypeStr=boolean
  Relational Operator1 : RelationalOperator  Operator=<  OutDataTypeStr=boolean
  Sinal_Pulso : Outport
  wires:
  Gain1/1 -> Add/2
  Theta/1 -> Add/1
  Add/1 -> Math Function/1
  Math Function/1 -> Relational Operator1/1, Relational Operator/1
  Relational Operator/1 -> Logical Operator/1
  Relational Operator1/1 -> Logical Operator/2
  Constant/1 -> Relational Operator/2
  Divide/1 -> Math Function/2, Gain/1, Gain1/1  "Theta_p"
  Gain/1 -> Relational Operator1/2
  Logical Operator/1 -> Sinal_Pulso/1
  Constant2/1 -> Divide/1
  Constant1/1 -> Divide/2

== system teste/Encoder1/Subsystem ==
  note: Dependendo do sentido da rotaçao, incrementa ou decrementa o contador
  POS : Inport
  NEG : Inport  Port=2
  Constant : Constant  Value=4*Nr
  Conversion : DataTypeConversion  OutDataTypeStr=int32
  Conversion1 : DataTypeConversion  OutDataTypeStr=int32
  Math Function : Math  Operator=mod  SaturateOnIntegerOverflow=on
  Memory : Memory
  Sum : Sum  Inputs=+-+
  Out : Outport
  wires:
  NEG/1 -> Conversion1/1
  Conversion1/1 -> Sum/2
  Conversion/1 -> Sum/1
  POS/1 -> Conversion/1
  Math Function/1 -> Memory/1
  Memory/1 -> Sum/3, Out/1
  Sum/1 -> Math Function/1

== system teste/M//T/Memória controlavel ==
  note: Memória controlável
      |
      | Se "ctrl" = 1, "Out" = "In"
      | Se "ctrl" = 0, "Out" mantém mesmo valor
  In : Inport
  ctrl : Inport  Port=2
  Memory2 : Memory
  Switch2 : Switch
  Out : Outport
  wires:
  Switch2/1 -> Memory2/1
  Memory2/1 -> Out/1, Switch2/3
  ctrl/1 -> Switch2/2
  In/1 -> Switch2/1

== system teste/M//T/Memória controlavel1 ==
  note: Memória controlável
      |
      | Se "ctrl" = 1, "Out" = "In"
      | Se "ctrl" = 0, "Out" mantém mesmo valor
  In : Inport
  ctrl : Inport  Port=2
  Memory2 : Memory
  Switch2 : Switch
  Out : Outport
  wires:
  In/1 -> Switch2/1
  ctrl/1 -> Switch2/2
  Memory2/1 -> Switch2/3, Out/1
  Switch2/1 -> Memory2/1

== system teste/M//T/Memória controlavel2 ==
  note: Memória controlável
      |
      | Se "ctrl" = 1, "Out" = "In"
      | Se "ctrl" = 0, "Out" mantém mesmo valor
  In : Inport
  ctrl : Inport  Port=2
  Memory2 : Memory
  Switch2 : Switch
  Out : Outport
  wires:
  In/1 -> Switch2/1
  ctrl/1 -> Switch2/2
  Memory2/1 -> Switch2/3, Out/1
  Switch2/1 -> Memory2/1
